simulink model "Transmitancje"  (R2018b)
settings: Solver=FixedStepAuto  StartTime=0.0  StopTime=50000  FixedStep=10  MaxStep=1  RelTol=1e-3
values from neighbouring files (symbols this model uses):
  dt = 500    [script1.m]
  dTg = 0    [script1.m]
  dTkz = 0    [script1.m]
  dTzew = 0    [script1.m]
  L11 = [Cp0*CVp, Cp0*(kp+k2)]    [script1.m]
  L12 = [CVp*k1, k1*(k2+kp)]    [script1.m]
  L13 = [k2*kp]    [script1.m]
  L21 = [Cp0*kp]    [script1.m]
  L22 = [k1*kp]    [script1.m]
  L23 = [CVw*k2 (k2*Cp0+k1*k2+k2*kp)]    [script1.m]
  M = [CVw * CVp, CVw*kp + CVw*k2 + Cp0*CVp + CVp*k1 + CVp*kp, (kp+k2)*(Cp0) + k1*kp + k1*k2 + kp*k2]    [script1.m]
  Tp0 = (kp * Twew0 + k2 * Tg0) / (k2 + kp)    (= 10)    [script1.m]
  Twew0 = (Cp0 * Tkz0 + k1 * Tzew0 + k2 * kp * Tg0 / (k2 + kp)) / (Cp0 + k1 + kp - kp * kp / (k2 + kp))    (= 20)    [script1.m]
settings Model: Creator=aplov  LastModifiedBy=wojciechkonury
settings DebuggingCC: LibraryContextMissingDiagnostic=none
settings SFSimCC: SimUseLocalCustomCode=off
settings RTWCC: RTWUseLocalCustomCode=off

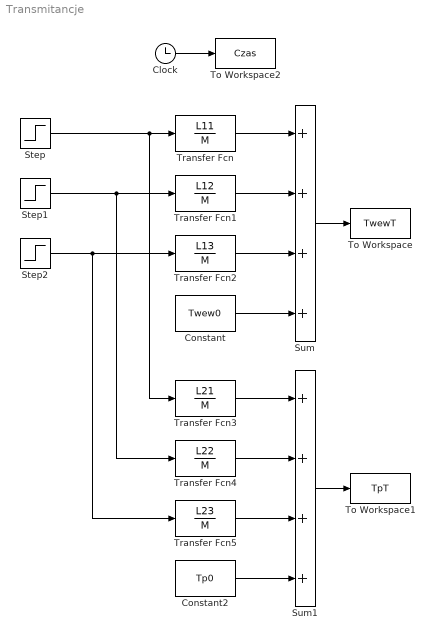
== system Transmitancje ==
  Clock : Clock
  Constant : Constant  Value=Twew0
  Constant2 : Constant  Value=Tp0
  Step : Step  Time=dt  After=dTkz  SampleTime=0
  Step1 : Step  Time=dt  After=dTzew  SampleTime=0
  Step2 : Step  Time=dt  After=dTg  SampleTime=0
  Sum : Sum  Inputs=++++
  Sum1 : Sum  Inputs=++++
  To Workspace : ToWorkspace  VariableName=TwewT  SampleTime=-1
  To Workspace1 : ToWorkspace  VariableName=TpT  SampleTime=-1
  To Workspace2 : ToWorkspace  VariableName=Czas  SampleTime=-1
  Transfer Fcn : TransferFcn  Numerator=L11  Denominator=M
  Transfer Fcn1 : TransferFcn  Numerator=L12  Denominator=M
  Transfer Fcn2 : TransferFcn  Numerator=L13  Denominator=M
  Transfer Fcn3 : TransferFcn  Numerator=L21  Denominator=M
  Transfer Fcn4 : TransferFcn  Numerator=L22  Denominator=M
  Transfer Fcn5 : TransferFcn  Numerator=L23  Denominator=M
  wires:
  Transfer Fcn/1 -> Sum/1
  Transfer Fcn1/1 -> Sum/2
  Transfer Fcn2/1 -> Sum/3
  Constant/1 -> Sum/4
  Transfer Fcn3/1 -> Sum1/1
  Transfer Fcn4/1 -> Sum1/2
  Transfer Fcn5/1 -> Sum1/3
  Constant2/1 -> Sum1/4
  Sum/1 -> To Workspace/1
  Sum1/1 -> To Workspace1/1
  Step/1 -> Transfer Fcn3/1, Transfer Fcn/1
  Step1/1 -> Transfer Fcn4/1, Transfer Fcn1/1
  Step2/1 -> Transfer Fcn5/1, Transfer Fcn2/1
  Clock/1 -> To Workspace2/1
